simulink model "foc"  (R2021a)
settings: Solver=VariableStepAuto  StartTime=0.0  StopTime=10.0  RelTol=1e-3
libraries: pspsim x1
settings Model: Creator=ahmet  LastModifiedBy=ahmet

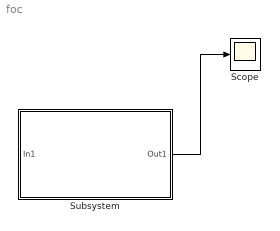
== system foc ==
  Scope : Scope
  Subsystem : Subsystem
  wires:
  Subsystem/1(Out1) -> Scope/1

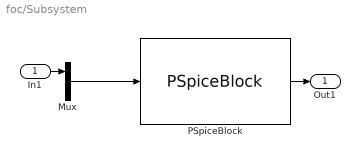
== system foc/Subsystem ==
  In1 : Inport
  Mux : Mux  Inputs=2
  PSpiceBlock : pspsim/PSpiceBlock  SFunctionModules=''
      settings: SourceProductName=PSpice Block
  Out1 : Outport
  wires:
  PSpiceBlock/1 -> Out1/1
  Mux/1 -> PSpiceBlock/1
  In1/1 -> Mux/1
